simulink model "hold3"  (R2018b)
settings: Solver=VariableStepAuto  StartTime=0.0  StopTime=10.0  RelTol=1e-3
settings Model: Creator=iamcy  LastModifiedBy=iamcy

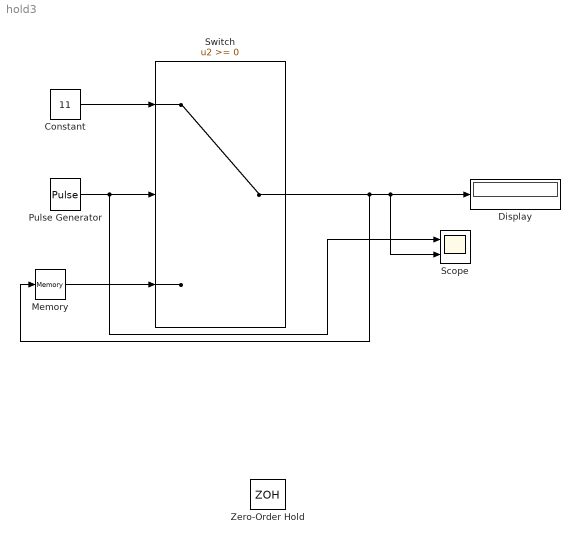
== system hold3 ==
  Constant : Constant  Value=11
  Display : Display
      settings: Decimation=2
  Memory : Memory
  Pulse Generator : DiscretePulseGenerator  PulseType=Time based  Period=13  PulseWidth=100/13
  Scope : Scope  NumInputPorts=2
  Switch : Switch
  Zero-Order Hold : ZeroOrderHold  SampleTime=-1
  wires:
  Memory/1 -> Switch/3
  Switch/1 -> Scope/2, Display/1, Memory/1
  Pulse Generator/1 -> Scope/1, Switch/2
  Constant/1 -> Switch/1
